simulink model "heater_stateflow"  (R2016a)
settings: Solver=FixedStepDiscrete  StartTime=0.0  StopTime=10.0  FixedStep=0.1  RelTol=1e-3
settings Model: Creator=zhanh  LastModifiedBy=zhanh
settings SolverCC: AutoInsertRateTranBlk=on
settings DataIOCC: LimitDataPoints=on
settings DebuggingCC: AllowSymbolicDim=off
settings ConfigComp: CovModelRefEnable=Off  CovSFcnEnable=off

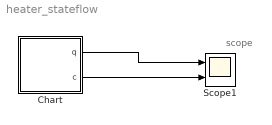
== system heater_stateflow ==
  note: scope
  Chart : Stateflow chart  TreatAsAtomicUnit=on
  Scope1 : Scope  NumInputPorts=2
  wires:
  Chart/1(q) -> Scope1/1
  Chart/2(c) -> Scope1/2

== stateflow chart heater_stateflow/Chart ==
  note: heater
  state heater
    during:
    c=c-0.026*(c-q);
    q=q+1;
  (default) -> heater : {c=73;q=73;}
  data: q output; c output
